simulink model "rounded_step_tesing_sim_bowen"  (R2023b)
settings: Solver=FixedStepAuto  StartTime=0.0  StopTime=10.0  FixedStep=0.01  RelTol=1e-3
undefined symbols (not defined in the file): stepp
settings Model: Creator=Nico  LastModifiedBy=dixiao
settings RTWCC: GPUComputeCapability=5.0
settings ConfigComp: CovBoundaryAbsTol=1.0e-5

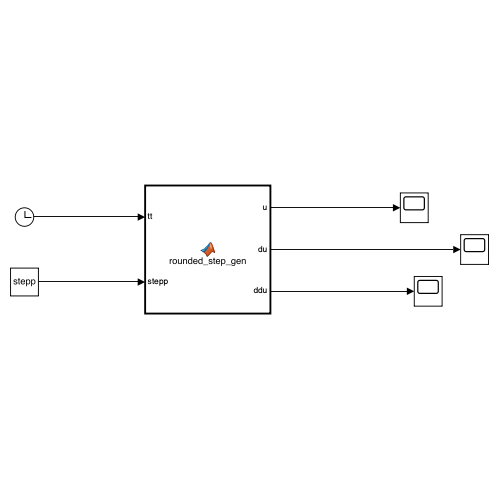
[thumbnail: Simulink's stored preview of the top-level diagram]
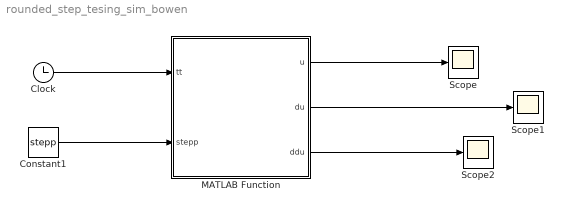
== system rounded_step_tesing_sim_bowen ==
  Clock : Clock
  Constant1 : Constant  Value=stepp
  MATLAB Function : MATLAB Function  TreatAsAtomicUnit=on
  Scope : Scope
  Scope1 : Scope
  Scope2 : Scope
  wires:
  Constant1/1 -> MATLAB Function/2(stepp)
  MATLAB Function/1(u) -> Scope/1
  MATLAB Function/2(du) -> Scope1/1
  MATLAB Function/3(ddu) -> Scope2/1
  Clock/1 -> MATLAB Function/1(tt)

== matlab function rounded_step_tesing_sim_bowen/MATLAB Function ==
  data: tt input; u output; stepp input; du output; ddu output
function [u,du,ddu] = rounded_step_gen(tt,stepp)
    %{
    Three input parameters are passed to this function in the
    list stepp, namely st0, t1 and t3, in this sequence.
    
    Function to generate a rounded unit step function of time, tt.
    If st0 is zero, the step is generated as starting with zero
    slope at time 0 and increasing with a parabolic curve until t1.
    Then it changes to increasing linearly with the same slope as
    that of the parabola at t1, until t2 (which is calculated by
    the function), after which it increases with negative second
    derivative, with the same parabolic shape, until it reaches the
    unit step function value at t3, with zero slope.  The slope of
    the curve is the same just before and just after t2.

    The whole rounded step can be delayed by st0.    
    %}
    st0 = stepp(1);t1 = stepp(2);t3 = stepp(3);
    alpha = 1/(t3 - t1)/t1/2;
    beta  = -alpha*t1*t1;
    t2    = t3 - t1;

    A = [t2, 1;t3, 1];
    b = [alpha*(t2*t2 + 2*t1*t2 - t1*t1);1 + alpha*t3*t3];

    x = A\b;
    gamma = x(1);
    eta   = x(2);

    st1 = st0 + t1;
    st2 = st0 + t2;
    st3 = st0 + t3;
    ta  = tt - st0;
    if tt <= st0
        u   = 0;
        du  = 0;
        ddu = 0;
    elseif tt <= st1
        u   = alpha*ta*ta;
        ddu = 2*alpha;
        du  = ddu*ta;
    elseif tt <= st2
        u   = 2*alpha*t1*ta + beta;
        du  = 2*alpha*t1;
        ddu = 0;
    elseif tt <= st3
        u   = -alpha*ta*ta + gamma*ta + eta;
        ddu = -2*alpha;
        du  = ddu*ta + gamma;
    else
        u  = 1;
        du  = 0;
        ddu = 0;
    end
end
